simulink model "simpleMicrogrid_v1"  (R2020a)
settings: Solver=VariableStepAuto  StartTime=0.0  StopTime=24*60*60  RelTol=1e0
values from neighbouring files (symbols this model uses):
  to = 0.1    [v2gdata.mat]
  V2G =     [v2gdata.mat]
undefined symbols (not defined in the file or in its folder): A, B, C, Dd, Init, j, sigbuilder_block
libraries: simulink x28, powerlib x27, powerlib_meascontrol x5, simulink_extras x5, sps_avr x1, spsDieselMotorModel x1
(part 1 of 2)
settings Model: SimulationMode=accelerator  Creator=jlesage  LastModifiedBy=marko
settings DataIOCC: ReturnWorkspaceOutputs=off
settings DebuggingCC: UnconnectedInputMsg=none  UnconnectedOutputMsg=none  UnconnectedLineMsg=none  ArithmeticOperatorsInVariantConditions=warning
settings SFSimCC: SimUseLocalCustomCode=off  CustomCodeUndefinedFunction=UseInterfaceOnly
settings RTWCC: RTWUseLocalCustomCode=off

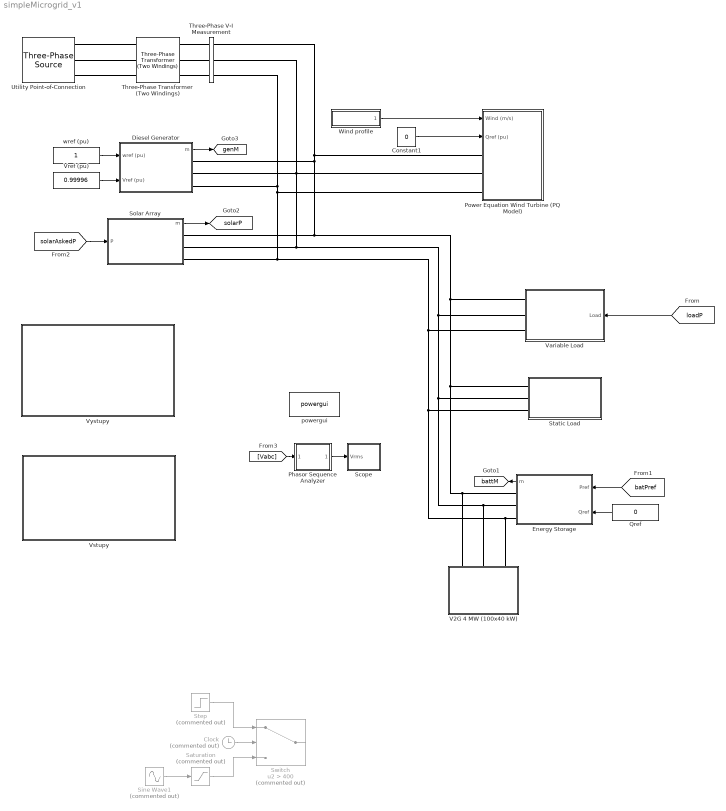
== system simpleMicrogrid_v1 ==
  Clock : Clock  Commented=on
  Constant1 : Constant  Value=0
  Diesel Generator : Subsystem  mask(Diesel Generator (Simple)){Pn=20e6, Vn=5000, Fn=60, genType=PQ, PQ0=[0.05 0]}
      mask prompts: Pn "Generator Rated Power [W]"; Vn "Rated Voltage [V]"; Fn "Rated Frequency [Hz]"; genType "Load Flow Type"; PQ0 "Initial Power, [P0 Q0] [pu]"
      mask help:
      | The Diesel Generator block contains a synchronous generator, diesel governor and excitation system to represent the dynamics of a Genset. To inspect the model, look under the block mask (Ctrl + u).
      |
      | The inputs to the basic Diesel generator block are the desired speed reference (in pu) and the desired voltage reference (in pu). The output measurements are contained in a Simulink bus, which can be selected by using the Bus Selector block.
      |
      | Note: The initial generator power must be specified for use for Load Flow analysis.
      mask init:
      | % Extract Initial Active/Reactive Power
      | P0 = PQ0(1);
      | Q0 = PQ0(2);
      | 
      | % Select Load Flow Type
      | genBlock = [gcb '/Synchronous Machine'];
      | currentVals = get_param(genBlock,'MaskValues');
      | currentVals{31} = genType;
      | set_param(genBlock,'MaskValues',currentVals);
      | 
      | % Disable Option if Swing Generator Selected
      | currentEnables = get_param(gcb,'MaskEnables');
      | if strcmp(genType,'swing')
      |     currentEnables{5} = 'off';
      | else
      |     currentEnables{5} = 'on';
      | end
      | set_param(gcb,'MaskEnables',currentEnables);
      settings: AttributesFormatString=Rated Power: %<Pn> W
      mask TypeOptions genType: swing | PQ | PV
      mask Display: %image(imread('diesel.jpg'))
  Energy Storage : Subsystem  mask(Grid-connected Energy Storage (PQ Model)){Vn=5000, Fn=60, PnomkW=5e5, kWh_Rated=1e5, Efficiency=96, LimitVec=[90 10], RechargeSOC=11, Precharge=50, autoRecharge=off, Initial_kWh_pc=80, PQvec=[100e3 0]}
      mask prompts: Vn "Nominal L-L Voltage [Vrms]"; Fn "Nominal Frequency [Hz]"; PnomkW "Rated Power [kW]"; kWh_Rated "Rated Capacity [kWh]"; Efficiency "Overall System Efficiency [%]"; LimitVec "Upper/Lower Charge Limits [%]"; RechargeSOC "SOC to Recharge [%]"; Precharge "Recharge Rate [% of Rated Power]"; autoRecharge "Enable Auto-Recharge"; Initial_kWh_pc "Initial State-of-Charge [0-100%]"; PQvec "Initial Active/Reactive Cmds"
      mask help:
      | The energy storage block models a generic grid-connected energy storage system (ESS), most commonly a battery system. This is a system-level model that does not contain any power electronics, but is useful for load flow, phasor, and hybrid phasor-EMT simulations. The inputs to this block are the commanded active and reactive power of the ESS. The ESS is assumed to have four quadrent operation.
      |
      | For more detailed ESS models, consider the battery block in the Drives library. Consider using this PQ Model to perform load flow studies and switch to a more detailed model when full EMT studies or more advanced controls are required.
      |
      | Note: The initial active/reactive power commands must be specified for use for Load Flow analysis.
      mask init:
      | % Calculate Initial Conditions
      | Pnom = PnomkW*1e3;
      | P0 = -PQvec(1);  Q0 = -PQvec(2);
      | if abs(P0) > Pnom
      |     P0 = sign(P0)*Pnom;
      | end
      | 
      | % Calculate Q0 given Reactive Power Capability Curve
      | Qlim = sqrt(Pnom^2 - P0^2);
      | if Qlim > abs(Q0)
      |     Q0 = sign(Q0)*Qlim;
      | end
      | 
      | UpChrgLim = LimitVec(1);
      | LowChrgLim = LimitVec(2);
      | if Initial_kWh_pc > UpChrgLim && P0 < 0
      |     P0 = 0; Q0 = 0;
      | elseif Initial_kWh_pc < LowChrgLim && P0 > 0
      |     P0 = 0; Q0 = 0;
      | end
      mask DialogControl Container7 Prompt: Grid Connection Properties
      mask DialogControl Container11 Prompt: Charge/Discharge Controls
      mask DialogControl Container12 Prompt: Initial Conditions
  Phasor Sequence Analyzer : Subsystem
  Power Equation Wind Turbine (PQ Model) : Subsystem  AncestorBlock=|  mask{Unom=15, Umax=25, Umin=5, Pselect=Simple Cubic Power, rp=5, Cp=16/27, rho=1.225, Pnom=500e3, Uvec=[1:1:30], Pvec=[0,0,0,0,21359.3750000000,58193.5000000000,104316.125000000,157104.500000000,213935.875000000,272187.500000000,329236.625000000,382460.500000000,429236.375000000,466941.500000000,492953.125000000,500000,500000,500000,500000,500000,500000,500000,500000,500000,500000,0,0,0,0,0], Tp=0.1, Tq=1, ReactP=30}
      | exampleMicrogridLibrary/Power Equation
      | Wind Turbine
      | (PQ Model)
      mask prompts: Unom "Nominal Wind Speed [m/s]"; Umax "Maximum Operating Wind [m/s]"; Umin "Minimum Operating Wind [m/s]"; Pselect "Wind Turbine Power Method"; rp "Blade Radius, r [m]"; Cp "Performance Coefficient, Cp"; rho "Air Density, rho [kg/m^3]"; Pnom "Nominal Power, [W]"; Uvec "Wind Vec [m/s]"; Pvec "Power Vec [W]"; Tp "Active Power Dynamics, Tp [s]"; Tq "Reactive Power Dynamics, Tq [s]"; ReactP "Reactive Power Percentage [%]"
      mask help:
      | Simple Wind Turbine that serves as an Active and Reactive Power Source depending on the Wind Power Curve.
      |
      | The Wind Turbine Power Curve can be defined by:
      | - Dimentions of the wind turbine
      | - Simple cubic power curve
      | - Look-up vector from a wind turbine data sheet.
      mask init:
      | A = pi*rp^2;
      | 
      | if Pselect == 1,
      |     Pmax = 1/2*rho*Cp*A*Umax^3;
      | elseif Pselect == 2,
      |     Pmax = Pnom;
      | else
      |     Pmax = max(Pvec);
      | end
      | Qmax = ReactP/100*Pmax;
      mask TypeOptions Pselect: Using Properties | Simple Cubic Power | Look-up Fit
      mask DialogControl Container4 Prompt: General
      mask DialogControl Container9 Prompt: Dimensions
      mask DialogControl Container12 Prompt: Cubic
      mask DialogControl Container7 Prompt: Lookup
      mask DialogControl Container8 Prompt: Dynamics
      mask Display:
      | image(imread('eolienne.bmp'))
      | 
      | color('white')
      | port_label('LConn',1,'A')
      | port_label('LConn',2,'B')
      | port_label('LConn',3,'C')
      | 
      | color('blue')
      | port_label('output',1,'m')
      | port_label('input',1,'Wind (m/s)')
      | port_label('input',2,'Qref')
  Qref : Constant  Value=0
  Saturation : Saturate  Commented=on  UpperLimit=15  LowerLimit=0
  Scope : Subsystem
  Sine Wave1 : Sin  Commented=on  Amplitude=20  Frequency=0.05  SampleTime=0
  Solar Array : Subsystem  mask(Grid-Connected PV Array (PQ Model)){Vn=5000, Fn=60, P0=500e3}
      mask prompts: Vn "Nominal L-L Voltage [Vrms]"; Fn "Nominal Frequency [Hz]"; P0 "Initial Power [W]"
      mask help:
      | This block models a grid-connected solar array using the Three-Phase Dynamic Load block. This is a system-level model that does not contain any power electronics, but is useful for load flow, phasor, and hybrid phasor-EMT simulations. The input to this block is the power output of the grid connected PV array, not irradiance.
      |
      | For more detailed PV models, consider the PV Array block in the Renewables library. Consider using this PQ Model to perform load flow studies and switch to a more detailed model when full EMT studies are required.
      |
      | Note: The array power must be specified for use for Load Flow analysis.
      mask init:
      | % P0 = Irr0*TotalArea*Efficiency/100;
      | P0 = -P0;
      mask Display:
      | image(imread('PV_Farm.jpg'))
      | color('white')
      | port_label('input',1,'P')
      | port_label('output',1,'m')
      | port_label('Rconn',1,'A')
      | port_label('Rconn',2,'B')
      | port_label('Rconn',3,'C')
  Static Load : Subsystem
  Step : Step  Commented=on  Time=550  Before=10  After=0  SampleTime=0
  Switch : Switch  Commented=on  Criteria=u2 > Threshold  Threshold=400
  Three-Phase Transformer (Two Windings) : powerlib/Elements/Three-Phase Transformer (Two Windings)  Winding1Connection=Yg  Winding2Connection=Yg  CoreType=Three single-phase transformers  SetSaturation=off  Hysteresis=off  DataFile='hysteresis'  SetInitialFlux=off  Measurements=None  UNITS=pu  NominalPower=[ 250e6 , 60 ]  Winding1=[ 13.8e3 , 0.002 , 0.08 ]  Winding2=[ 5000 , 0.002 , 0.08 ]  Rm=500  Lm=500  L0=0.5  Saturation=[ 0,0 ; 0.0024,1.2 ; 1.0,1.52 ]  InitialFluxes=[ 0.8 , -0.8 , 0.7 ]  BreakLoop=off  DiscreteSolver=Trapezoidal iterative  DataType=off  TransfoNumber=1
  Three-Phase V-I Measurement : powerlib/Measurements/Three-Phase V-I Measurement  VoltageMeasurement=phase-to-ground  SetLabelV=on  LabelV=Vabc  Vpu=off  VpuLL=off  CurrentMeasurement=yes  SetLabelI=on  LabelI=Iabc  Ipu=off  Pbase=100e6  Vbase=500e3  OutputType=Complex  PhasorSimulation=on  PSBequivalent=0
  Utility Point-of-Connection : powerlib/Electrical Sources/Three-Phase Source  InternalConnection=Yg  VoltagePhases=off  Voltage=(13800)*1.00293  PhaseAngle=0.16496  Voltage_phases=[25e3 25e3 25e3]/sqrt(3)  PhaseAngles_phases=[0 -120 +120]  Frequency=60  NonIdealSource=on  SpecifyImpedance=on  Resistance=0.8929  Inductance=16.58e-3  ShortCircuitLevel=250e6  BaseVoltage=13.8e3  XRratio=7  BusType=swing  Pref=10e3  Qref=0  Prefabc=[10e3, 10e3, 10e3]  Qrefabc=[0, 0, 0]  Qmin=-inf  Qmax=inf
  V2G 4 MW (100x40 kW) : Subsystem  mask{nomPower=20*2, capacity=85, eff=90, enable=on, regGain=[2 4e3], cars1=4, cars2=3, cars3=3, cars4=2, cars5=1}
      mask prompts: nomPower "Rated power (kW)"; capacity "Rated capacity (kWh)"; eff "System efficiency (%)"; enable "V2G on"; regGain "Regulator gain [Kp Ki]"; cars1 "Number of cars  (profile 1)"; cars2 "Number of cars  (profile 2)"; cars3 "Number of cars  (profile 3)"; cars4 "Number of cars  (profile 4)"; cars5 "Number of cars  (profile 5)"
      mask DialogControl DescGroupVar Prompt: V2G
      mask DialogControl DescTextVar Prompt: Models a generic aggregation of electric vehicles. The model has 5 different profiles that can be modified under the mask by changing the plug and the state of charge lookup tables of each profile. The user can set the number of vehicles following each type of profile. The rated capacity, the rated power and the efficiency of the power converter can also be decided by the user. See the example documentation for information about various user profiles.
      mask Display: image(imread('EV.jpg'))
  Variable Load : Subsystem  mask(Variable Load (PQ Model)){Vn=5000, Fn=60, PF=0.9500, Load0=200e3}
      mask prompts: Vn "Nominal L-L Voltage [Vrms]"; Fn "Nominal Frequency [Hz]"; PF "Power Factor [0 to 1]"; Load0 "Initial Load [W]"
      mask help:
      | The Variable Load block is a lumped approximation for a distribution feeder. For non-unity power factor loads, the input (active power) is scaled accordingly to generate a desired load.
      |
      | Note: The initial input load must be specified for use for Load Flow analysis.
      mask init:
      | P0 = Load0;
      | Q0 = Load0*sqrt(1/PF-1);
      mask Display:
      | image(imread('Residential.jpg'))
      | color('white')
      | port_label('input',1,'Load')
      | port_label('Rconn',1,'A')
      | port_label('Rconn',2,'B')
      | port_label('Rconn',3,'C')
  Vref (pu) : Constant  Value=0.99996
  Vstupy : Subsystem
  Vystupy : Subsystem
  Wind profile : Subsystem
      mask init:
      | load power_V2G
      mask Display: plot(V2G.WINDTURBINE.time,V2G.WINDTURBINE.wind)
  powergui : powerlib/powergui  Priority=1  SimulationMode=Phasor  SampleTime=1e-4  frequency=60  Iterations=50  frequencyindice=60  Pbase=100e6  ErrMax=1e-08  UnitsV=kV  UnitsW=MW  buscounter=6  FunctionMessages=off  echomessages=off  EnableUseOfTLC=off  CurrentSourceSwitches=off  DisableSnubberDevices=off  DisableRonSwitches=off  DisableVfSwitches=off  DisplayEquations=off  AutomaticDiscreteSolvers=off  SolverType=Tustin/Backward Euler (TBE)  Interpol=off  ExternalGateDelay=off  methode=off  Ts=100  x0status=blocks  SPID=on  SwTol=0  HookPort=off  NonlinearTolerance=1e-4  nMaxIteration=100  ContinueOnMaxIteration=off  RestoreLinks=warning  ResistiveCurrentMeasurement=off  Frange=[0:2:500]  Ylog=off  Xlog=on  ShowGrid=off  save=off  variable=ZData  structure=0  ZoomFFT=off  StartTime=0.0  cycles=1  DisplayStyle=1  fundamental=60  FreqAxis=off  MaxFrequency=1000  frequencyindicesteady=1  RmsSteady=1  display=off
  wref (pu) : Constant
  tag scope: battM=global, genM=global, solarP=global
  wires:
  Qref/1 -> Energy Storage/2(Qref)
  Energy Storage/1(m) -> [battM]
  Phasor Sequence Analyzer/1(Vrms) -> Scope/1(Vrms)
  [Vabc] -> Phasor Sequence Analyzer/1(Vabc)
  Step/1 -> Switch/1
  Sine Wave1/1 -> Saturation/1
  Saturation/1 -> Switch/3
  Clock/1 -> Switch/2
  wref (pu)/1 -> Diesel Generator/1(wref (pu))
  Diesel Generator/1(m) -> [genM]
  Vref (pu)/1 -> Diesel Generator/2(Vref (pu))
  Solar Array/1(m) -> [solarP]
  Wind profile/1(" ") -> Power Equation Wind Turbine (PQ Model)/1(Wind (m/s))
  Constant1/1 -> Power Equation Wind Turbine (PQ Model)/2(Qref (pu))
  [loadP] -> Variable Load/1(Load)
  [solarAskedP] -> Solar Array/1(P)
  [batPref] -> Energy Storage/1(Pref)
  connections:
  Diesel Generator/RConn2 -- Static Load/LConn2 -- Energy Storage/RConn2 -- V2G 4 MW (100x40 kW)/LConn2 -- Variable Load/RConn2 -- Solar Array/RConn2 -- Power Equation Wind Turbine (PQ Model)/LConn2 -- Three-Phase V-I Measurement/RConn2
  Energy Storage/RConn1 -- V2G 4 MW (100x40 kW)/LConn1 -- Static Load/LConn1 -- Variable Load/RConn1 -- Three-Phase V-I Measurement/RConn1 -- Power Equation Wind Turbine (PQ Model)/LConn1 -- Diesel Generator/RConn1 -- Solar Array/RConn1
  Energy Storage/RConn3 -- V2G 4 MW (100x40 kW)/LConn3 -- Static Load/LConn3 -- Variable Load/RConn3 -- Solar Array/RConn3 -- Three-Phase V-I Measurement/RConn3 -- Diesel Generator/RConn3 -- Power Equation Wind Turbine (PQ Model)/LConn3
  Three-Phase Transformer (Two Windings)/RConn3 -- Three-Phase V-I Measurement/LConn3
  Three-Phase Transformer (Two Windings)/RConn2 -- Three-Phase V-I Measurement/LConn2
  Three-Phase Transformer (Two Windings)/RConn1 -- Three-Phase V-I Measurement/LConn1
  Utility Point-of-Connection/RConn1 -- Three-Phase Transformer (Two Windings)/LConn1
  Utility Point-of-Connection/RConn2 -- Three-Phase Transformer (Two Windings)/LConn2
  Utility Point-of-Connection/RConn3 -- Three-Phase Transformer (Two Windings)/LConn3

== system simpleMicrogrid_v1/Diesel Generator ==
  wref (pu) : Inport
  Vref (pu) : Inport  Port=2
  AC1A Excitation System : sps_avr/AC1A Excitation System  Tr=20e-3  KaTa=[400 0.02]  VAminmax=[-14.5 14.5]  VRminmax=[-5.43 6.03]  KfTf=[0.03 1.0]  TbTc=[0 0]  KeTe=[1.0 0.80]  Ve12=[4.18 3.14]  SeVe12=[0.10 0.03]  Kd=0.38  Kc=0.20  v0=[0.99996 1.0014]  TsBlock=0
      settings: SourceProductBaseCode=PS
  Diesel Engine Governor : spsDieselMotorModel/Diesel Engine Governor  K=29  Tr=[0.01 0.02 0.2]  Ta=[0.25 0.009 0.0384]  Tlim=[0 1.1]  Td=0.024  Pm0=0.050008
      settings: SourceProductBaseCode=PS
  Generator Measures : Subsystem
  Ground : Ground
  Selected Measurements : Subsystem
  Synchronous Machine : powerlib/Machines/Synchronous Machine pu Standard  PresetModel=No  MechanicalLoad=Mechanical power Pm  ShowDetailedParameters=on  RotorType=Salient-pole  Units=per unit standard parameters  MeasurementBus=off  NominalParameters=[ Pn Vn Fn]  Reactances1=[ 1.81, 0.3, 0.23, 1.76, 0.65, 0.25, 0.15 ]  Reactances2="[ 1.305, 0.296, 0.252, 0.474,  0.243,  0.18 ]"  dAxisTimeConstants=Open-circuit  qAxisTimeConstants=Short-circuit  TimeConstants1="[ 4.4849  0.0681  0.1  ]"  TimeConstants2=[ 8.0, 0.03, 1.0, 0.07 ]  TimeConstants3="[  4.49  0.0681  0.0513  ]"  TimeConstants4=[ 8.0, 0.03, 0.3371, 0.0295 ]  TimeConstants5=[ 1.01, 0.053, 0.1 ]  TimeConstants6=[ 1.3201, 0.023, 1.0, 0.07 ]  TimeConstants7=[0.012 0.003 0.003]  TimeConstants8=[ 1.3201, 0.0231, 0.3371, 0.0295 ]  StatorResistance=0.003  Mechanical=[3.7 0 1 ]  PolePairs=20  InitialConditions=[0 -88.6613 0.0500019 0.0500019 0.0500019 -0.018842 -120.019 119.981 1.00138]  SetSaturation=off  Saturation=[0.6404,0.7127,0.8441,0.9214,0.9956,1.082,1.19,1.316,1.457;0.7,0.7698,0.8872,0.9466,0.9969,1.046,1.1,1.151,1.201]  LoadFlowParameters=[1,0,0,0,0]  TsPowergui=0  TsBlock=-1  IterativeModel=Trapezoidal non iterative  IterativeDiscreteModel=Trapezoidal non iterative  BusType=PQ  Pref=Pn*P0  Qref=0  Qmin=-inf  Qmax=inf  PLF=0  QLF=0
  A : PMIOPort  Side=Right
  B : PMIOPort  Port=2  Side=Right
  C : PMIOPort  Port=3  Side=Right
  m : Outport  VectorParamsAs1DForOutWhenUnconnected=off
  wires:
  wref (pu)/1 -> Diesel Engine Governor/1
  Vref (pu)/1 -> AC1A Excitation System/1
  Synchronous Machine/1 -> Generator Measures/1(m), Selected Measurements/1(m)
  Ground/1 -> AC1A Excitation System/4
  Generator Measures/3(wm) -> Diesel Engine Governor/2
  Generator Measures/2(Vt) -> AC1A Excitation System/2
  Generator Measures/1(Ifd) -> AC1A Excitation System/3
  Selected Measurements/1(sm) -> m/1
  Diesel Engine Governor/1 -> Synchronous Machine/1
  AC1A Excitation System/1 -> Synchronous Machine/2
  connections:
  Synchronous Machine/RConn1 -- A/RConn1
  Synchronous Machine/RConn3 -- C/RConn1
  Synchronous Machine/RConn2 -- B/RConn1

== system simpleMicrogrid_v1/Energy Storage ==
  Pref : Inport
  Qref : Inport  Port=2
  Bus Creator : BusCreator  Inputs=3
  Charge Limits : Subsystem
  Mux1 : Mux  Inputs=2
  Power Limits : Saturate  UpperLimit=Pnom  LowerLimit=-Pnom
  Reactive Power Capability : Subsystem
  Simple Battery Inverter : powerlib/Elements/Three-Phase Dynamic Load  NominalVoltage=[Vn Fn]  ActiveReactivePowers=[-100000 -3.07049e-13]  PositiveSequence=[0.999962 -0.018842]  ExternalControl=on  NpNq=[1.3 2]  TimeConstants="[0  0  0  0]"  MinimumVoltage=0.7  Tfilter=1e-2  LoadFlowParameters=[4,0,0,0,0]
      settings: SourceProductBaseCode=PS
  Stored Energy Calculation (%) : Subsystem
  Terminator : Terminator
  Unary Minus : UnaryMinus
  A : PMIOPort  Side=Right
  B : PMIOPort  Port=2  Side=Right
  C : PMIOPort  Port=3  Side=Right
  m : Outport  VectorParamsAs1DForOutWhenUnconnected=off
  wires:
  Charge Limits/2(Qbatt) -> Reactive Power Capability/2(Qin)
  Qref/1 -> Charge Limits/3(Qin)
  Power Limits/1 -> Charge Limits/2(Pin)
  Charge Limits/1(Pbatt) -> Reactive Power Capability/1(Pin), Unary Minus/1, Bus Creator/2, Stored Energy Calculation (%)/1(Pin)  "Pbatt"
  Stored Energy Calculation (%)/1(SE%) -> Bus Creator/1, Charge Limits/1(SOC (%))  "SOC (%)"
  Bus Creator/1 -> m/1
  Pref/1 -> Power Limits/1
  Reactive Power Capability/1(Qout) -> Mux1/2, Bus Creator/3, Stored Energy Calculation (%)/2(Qin)  "Qbatt"
  Simple Battery Inverter/1 -> Terminator/1
  Mux1/1 -> Simple Battery Inverter/1
  Unary Minus/1 -> Mux1/1
  connections:
  Simple Battery Inverter/LConn1 -- A/RConn1
  Simple Battery Inverter/LConn3 -- C/RConn1
  Simple Battery Inverter/LConn2 -- B/RConn1

== system simpleMicrogrid_v1/Phasor Sequence Analyzer ==
  Vabc : Inport
  Sequence Analyzer (Phasor) : powerlib_meascontrol/Measurements/Sequence Analyzer (Phasor)  seq=Positive
      settings: SourceProductBaseCode=PS
  Terminator : Terminator
  Vrms : Outport  VectorParamsAs1DForOutWhenUnconnected=off
  wires:
  Sequence Analyzer (Phasor)/1 -> Vrms/1
  Vabc/1 -> Sequence Analyzer (Phasor)/1
  Sequence Analyzer (Phasor)/2 -> Terminator/1

== system simpleMicrogrid_v1/Power Equation Wind Turbine (PQ Model) ==
  Wind (m/s) : Inport
  Qref (pu) : Inport  Port=2
  Active Power Dynamics : Subsystem  VariantControl=T6NotZero
      mask Display: disp('1 / (1 + s T_P)','texmode','on');
  Bus Selector : BusSelector  OutputSignals=Active power P (W)
  Ground : powerlib/Elements/Ground  LConnTagsString=a
  Mux : Mux  Inputs=2
  Reactive Power Dynamics : Subsystem  VariantControl=T6NotZero
      mask Display: disp('1 / (1 + s T_Q)','texmode','on');
  Saturation : Saturate  UpperLimit=Qmax  LowerLimit=-Qmax
  Scope1 : Scope
  Shunt (Numerical Stability) : powerlib/Elements/Three-Phase Series RLC Branch  LConnTagsString=A|B|C  RConnTagsString=A|B|C  BranchType=R  Resistance=1e9  Inductance=1e-3  Capacitance=1e-6  Measurements=None
  Three-Phase Dynamic Load : powerlib/Elements/Three-Phase Dynamic Load  NominalVoltage=[5000 60]  ActiveReactivePowers=[50e6 25e6]  PositiveSequence=[0.994 -11.8]  ExternalControl=on  NpNq=[1.3 2]  TimeConstants="[0  0  0  0]"  MinimumVoltage=0.7  Tfilter=1e-4  LoadFlowParameters=[4,0,0,0,0]
      settings: SourceProductBaseCode=PS
  Wind Turbine Power Equation : Subsystem
  A : PMIOPort  Side=Left
  B : PMIOPort  Port=2  Side=Left
  C : PMIOPort  Port=3  Side=Left
  tag scope: windP=global
  wires:
  Qref (pu)/1 -> Saturation/1
  Saturation/1 -> Reactive Power Dynamics/1(In)
  Reactive Power Dynamics/1(Out) -> Mux/2
  Active Power Dynamics/1(Out) -> Mux/1
  Mux/1 -> Three-Phase Dynamic Load/1
  Wind Turbine Power Equation/1(Pwind) -> Active Power Dynamics/1(In)
  Wind (m/s)/1 -> Wind Turbine Power Equation/1(Wind (m/s))
  Bus Selector/1 -> Scope1/1, [windP]  "<Active power P (W)>"
  Three-Phase Dynamic Load/1 -> Bus Selector/1
  connections:
  Ground/LConn1 -- Shunt (Numerical Stability)/RConn1 -- Shunt (Numerical Stability)/RConn2 -- Shunt (Numerical Stability)/RConn3
  Shunt (Numerical Stability)/LConn1 -- Three-Phase Dynamic Load/LConn1 -- A/RConn1
  Shunt (Numerical Stability)/LConn3 -- Three-Phase Dynamic Load/LConn3 -- C/RConn1
  Shunt (Numerical Stability)/LConn2 -- Three-Phase Dynamic Load/LConn2 -- B/RConn1

== system simpleMicrogrid_v1/Scope ==
  Vrms : Inport
  Bus Selector1 : BusSelector  OutputSignals=SOC (%)  OutputAsBus=on
  Bus Selector2 : BusSelector  OutputSignals=Pbatt
  Bus Selector3 : BusSelector  OutputSignals=Active Power (W)
  Bus Selector4 : BusSelector  OutputSignals="Rotor speed  wm  (pu)"
  Gain : Gain  Gain=60
  LG to LL : Gain  Gain=sqrt(3)/sqrt(2)
  Microgrid Measures : Scope  NumInputPorts=4
  Mux : Mux
  Scope : Scope
  to kW : Gain  Gain=1e-3
  wires:
  Bus Selector3/1 -> Mux/4  "<Active Power (W)>"
  to kW/1 -> Scope/1, Microgrid Measures/2  "Distributed Resources (kW)"
  Bus Selector4/1 -> Gain/1  "<Rotor speed  wm  (pu)>"
  [genM] -> Bus Selector4/1
  Gain/1 -> Microgrid Measures/1  "Microgrid Frequency (Hz)"
  Bus Selector1/1 -> Microgrid Measures/3  "Battery SOC (%)"
  [battM] -> Bus Selector1/1
  [genM] -> Bus Selector3/1
  [battM] -> Bus Selector2/1
  Bus Selector2/1 -> Mux/3  "<Pbatt>"
  [solarP] -> Mux/2
  Mux/1 -> to kW/1
  LG to LL/1 -> Microgrid Measures/4  "Microgrid Voltage (Vrms)"
  Vrms/1 -> LG to LL/1
  [windP] -> Mux/1

== system simpleMicrogrid_v1/Solar Array ==
  P : Inport
  Bus Selector : BusSelector  OutputSignals=Active power P (W)
  Constant11 : Constant  Value=0
  Mux1 : Mux  Inputs=2
  Simple Solar Inverter : powerlib/Elements/Three-Phase Dynamic Load  NominalVoltage=[Vn Fn]  ActiveReactivePowers=[-250000 -2.85874e-13]  PositiveSequence=[0.999962 -0.018842]  ExternalControl=on  NpNq=[1.3 2]  TimeConstants="[0  0  0  0]"  MinimumVoltage=0.7  Tfilter=1e-2  LoadFlowParameters=[4,0,0,0,0]
      settings: SourceProductBaseCode=PS
  Unary Minus : UnaryMinus
  Unary Minus1 : UnaryMinus
  A : PMIOPort  Side=Right
  B : PMIOPort  Port=2  Side=Right
  C : PMIOPort  Port=3  Side=Right
  m : Outport  VectorParamsAs1DForOutWhenUnconnected=off
  wires:
  P/1 -> Unary Minus/1
  Unary Minus/1 -> Mux1/1
  Constant11/1 -> Mux1/2
  Simple Solar Inverter/1 -> Bus Selector/1
  Bus Selector/1 -> Unary Minus1/1  "<Active power P (W)>"
  Unary Minus1/1 -> m/1
  Mux1/1 -> Simple Solar Inverter/1
  connections:
  Simple Solar Inverter/LConn2 -- B/RConn1
  Simple Solar Inverter/LConn3 -- C/RConn1
  Simple Solar Inverter/LConn1 -- A/RConn1

== system simpleMicrogrid_v1/Static Load ==
  Load : powerlib/Elements/Three-Phase Series RLC Load  LConnTagsString=A|B|C  Configuration=Y (grounded)  NominalVoltage=(5000)*0.999962  Vabc=[1e3 1e3 1e3]  Vabcp=[1e3 1e3 1e3]  NominalFrequency=60  UnbalancedPower=off  ActivePower=500e3  InductivePower=0  CapacitivePower=0  Pabc=[10e3 9e3 11e3]  QLabc=[100 90 110]  QCabc=[100 90 110]  Pabcp=[10e3 9e3 11e3]  QLabcp=[100 90 110]  QCabcp=[100 90 110]  Measurements=Branch voltages  LoadType=constant PQ
      settings: AttributesFormatString=P = %<ActivePower> W
  "Power (3ph, Phasor)5" : powerlib_meascontrol/Measurements/Power (3ph, Phasor)
      settings: SourceProductBaseCode=MT,PS
  Scope : Scope
  Terminator : Terminator
  Three-Phase V-I Measurement : powerlib/Measurements/Three-Phase V-I Measurement  VoltageMeasurement=phase-to-ground  SetLabelV=on  LabelV=VabcLoad  Vpu=off  VpuLL=off  CurrentMeasurement=yes  SetLabelI=on  LabelI=IabcLoad  Ipu=off  Pbase=100e6  Vbase=500e3  OutputType=Complex  PhasorSimulation=on  PSBequivalent=0
  A : PMIOPort  Side=Left
  B : PMIOPort  Port=2  Side=Left
  C : PMIOPort  Port=3  Side=Left
  tag scope: PLoad=global
  wires:
  [VabcLoad] -> "Power (3ph, Phasor)5"/1
  [IabcLoad] -> "Power (3ph, Phasor)5"/2
  "Power (3ph, Phasor)5"/2 -> Terminator/1  "Q(VA)"
  "Power (3ph, Phasor)5"/1 -> Scope/1, [PLoad]  "P(W)"
  connections:
  Load/LConn1 -- Three-Phase V-I Measurement/RConn1
  Load/LConn2 -- Three-Phase V-I Measurement/RConn2
  Load/LConn3 -- Three-Phase V-I Measurement/RConn3
  Three-Phase V-I Measurement/LConn1 -- A/RConn1
  B/RConn1 -- Three-Phase V-I Measurement/LConn2
  Three-Phase V-I Measurement/LConn3 -- C/RConn1

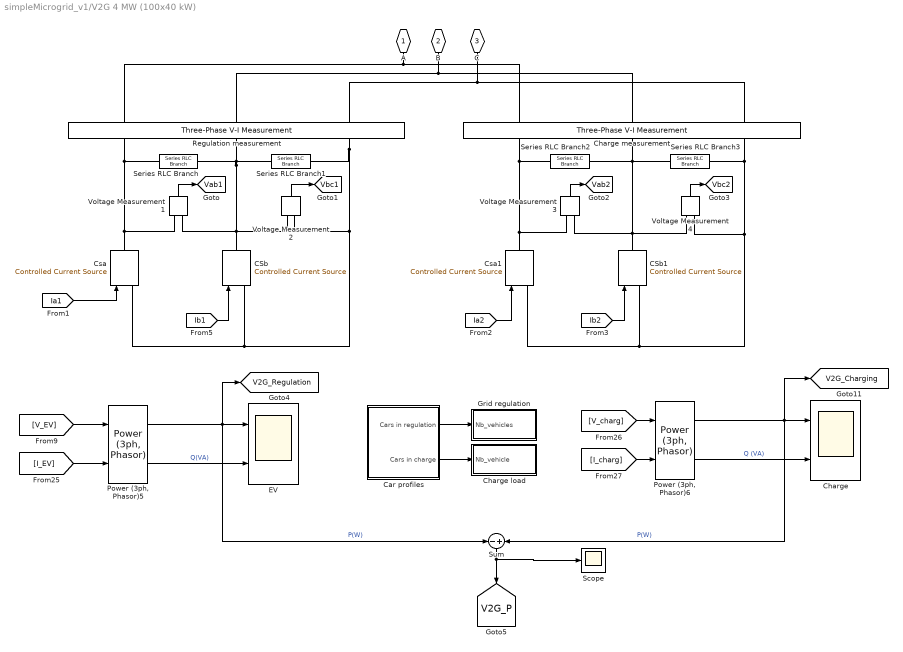
== system simpleMicrogrid_v1/V2G 4 MW (100x40 kW) ==
  " Charge measurement" : powerlib/Measurements/Three-Phase V-I Measurement  VoltageMeasurement=phase-to-ground  SetLabelV=on  LabelV=V_charg  Vpu=off  VpuLL=off  CurrentMeasurement=yes  SetLabelI=on  LabelI=I_charg  Ipu=off  Pbase=2*1.5e6/0.9  Vbase=25e3  OutputType=Complex  PhasorSimulation=on  PSBequivalent=0
      settings: SourceProductBaseCode=MT,PS
  " Regulation measurement" : powerlib/Measurements/Three-Phase V-I Measurement  VoltageMeasurement=phase-to-ground  SetLabelV=on  LabelV=V_EV  Vpu=off  VpuLL=off  CurrentMeasurement=yes  SetLabelI=on  LabelI=I_EV  Ipu=off  Pbase=2*1.5e6/0.9  Vbase=25e3  OutputType=Complex  PhasorSimulation=on  PSBequivalent=0
      settings: SourceProductBaseCode=MT,PS
  CSb : powerlib/Electrical Sources/Controlled Current Source  Initialize=on  Source_Type=AC  Amplitude=5604.181  Phase=(2.761-2*pi/3)*180/pi  Frequency=60  Measurements=Current
      settings: SourceProductBaseCode=MT,PS
  CSb1 : powerlib/Electrical Sources/Controlled Current Source  Initialize=on  Source_Type=AC  Amplitude=5604.181  Phase=(2.761-2*pi/3)*180/pi  Frequency=60  Measurements=Current
      settings: SourceProductBaseCode=MT,PS
  Car profiles : Subsystem
  Charge : Scope  NumInputPorts=2
  Charge load : Subsystem
  Csa : powerlib/Electrical Sources/Controlled Current Source  Initialize=on  Source_Type=AC  Amplitude=5604.181  Phase=2.761*180/pi  Frequency=60  Measurements=Current
      settings: SourceProductBaseCode=MT,PS
  Csa1 : powerlib/Electrical Sources/Controlled Current Source  Initialize=on  Source_Type=AC  Amplitude=5604.181  Phase=2.761*180/pi  Frequency=60  Measurements=Current
      settings: SourceProductBaseCode=MT,PS
  EV : Scope  NumInputPorts=2
  Grid regulation : Subsystem
  "Power (3ph, Phasor)5" : powerlib_meascontrol/Measurements/Power (3ph, Phasor)
      settings: SourceProductBaseCode=MT,PS
  "Power (3ph, Phasor)6" : powerlib_meascontrol/Measurements/Power (3ph, Phasor)
      settings: SourceProductBaseCode=MT,PS
  Scope : Scope
  Series RLC Branch{,1..3} (4 alike) : powerlib/Elements/Series RLC Branch  LConnTagsString=__new0  RConnTagsString=__new0  BranchType=R  Resistance=1e6  Inductance=1e-3  SetiL0=off  InitialCurrent=0  Capacitance=1e-6  Setx0=off  InitialVoltage=0  Measurements=None
      settings: SourceProductBaseCode=MT,PS
  Sum : Sum  Inputs=-+
  Voltage Measurement{1..4} (4 alike) : powerlib/Measurements/Voltage Measurement  PhasorSimulation=on  OutputType=Complex  PSBequivalent=0
      settings: SourceProductBaseCode=MT,PS
  "A " : PMIOPort  Tag=PMCPort  Side=Left
  B : PMIOPort  Tag=PMCPort  Port=2  Side=Left
  "C " : PMIOPort  Tag=PMCPort  Port=3  Side=Left
  tag scope: V2G_Charging=global, V2G_P=global, V2G_Regulation=global, Vab1=global, Vab2=global, Vbc1=global, Vbc2=global
  wires:
  Voltage Measurement1/1 -> [Vab1]
  Voltage Measurement2/1 -> [Vbc1]
  [Ia1] -> Csa/1
  [Ib1] -> CSb/1
  Voltage Measurement3/1 -> [Vab2]
  Voltage Measurement4/1 -> [Vbc2]
  [Ia2] -> Csa1/1
  [Ib2] -> CSb1/1
  Car profiles/1(Cars in regulation) -> Grid regulation/1(Nb_vehicles)
  Car profiles/2(" Cars in charge") -> Charge load/1(Nb_vehicle)
  [I_EV] -> "Power (3ph, Phasor)5"/2
  [V_charg] -> "Power (3ph, Phasor)6"/1
  [I_charg] -> "Power (3ph, Phasor)6"/2
  [V_EV] -> "Power (3ph, Phasor)5"/1
  "Power (3ph, Phasor)6"/1 -> Sum/2, [V2G_Charging], Charge/1  "P(W)"
  "Power (3ph, Phasor)6"/2 -> Charge/2  "Q (VA)"
  "Power (3ph, Phasor)5"/1 -> Sum/1, [V2G_Regulation], EV/1  "P(W)"
  "Power (3ph, Phasor)5"/2 -> EV/2  "Q(VA)"
  Sum/1 -> Scope/1, [V2G_P]
  connections:
  Series RLC Branch/LConn1 -- Csa/RConn1 -- Voltage Measurement1/LConn1 -- " Regulation measurement"/LConn1
  Voltage Measurement2/LConn2 -- Series RLC Branch1/RConn1 -- " Regulation measurement"/LConn3 -- Csa/LConn1 -- CSb/LConn1
  Voltage Measurement1/LConn2 -- " Regulation measurement"/LConn2 -- Series RLC Branch1/LConn1 -- Series RLC Branch/RConn1 -- CSb/RConn1 -- Voltage Measurement2/LConn1
  Voltage Measurement3/LConn1 -- Csa1/RConn1 -- Series RLC Branch2/LConn1 -- " Charge measurement"/RConn1
  Series RLC Branch3/RConn1 -- Csa1/LConn1 -- CSb1/LConn1 -- Voltage Measurement4/LConn2 -- " Charge measurement"/RConn3
  Series RLC Branch3/LConn1 -- Series RLC Branch2/RConn1 -- CSb1/RConn1 -- Voltage Measurement4/LConn1 -- Voltage Measurement3/LConn2 -- " Charge measurement"/RConn2
  " Regulation measurement"/RConn1 -- " Charge measurement"/LConn1 -- "A "/RConn1
  " Regulation measurement"/RConn2 -- " Charge measurement"/LConn2 -- B/RConn1
  " Regulation measurement"/RConn3 -- " Charge measurement"/LConn3 -- "C "/RConn1

== system simpleMicrogrid_v1/Variable Load ==
  Load : Inport
  Bus Selector : BusSelector  OutputSignals=Active power P (W)
  Dynamic Load Control : Subsystem
  Scope : Scope
  Simple Three-Phase Load : powerlib/Elements/Three-Phase Dynamic Load  NominalVoltage=[Vn Fn]  ActiveReactivePowers=[200000 45883.1]  PositiveSequence=[0.999962 -0.018842]  ExternalControl=on  NpNq=[1.3 2]  TimeConstants="[0  0  0  0]"  MinimumVoltage=0.7  Tfilter=1e-2  LoadFlowParameters=[4,0,0,0,0]
      settings: SourceProductBaseCode=PS
  A : PMIOPort  Side=Right
  B : PMIOPort  Port=2  Side=Right
  C : PMIOPort  Port=3  Side=Right
  tag scope: varLoadP=global
  wires:
  Simple Three-Phase Load/1 -> Bus Selector/1
  Load/1 -> Dynamic Load Control/1(P0)
  Dynamic Load Control/1(PQ) -> Scope/1, Simple Three-Phase Load/1
  Bus Selector/1 -> [varLoadP]  "<Active power P (W)>"
  connections:
  Simple Three-Phase Load/LConn1 -- A/RConn1
  Simple Three-Phase Load/LConn3 -- C/RConn1
  Simple Three-Phase Load/LConn2 -- B/RConn1

== system simpleMicrogrid_v1/Vstupy ==
  Add : Sum
  Bateria : Subsystem  Tag=STV Subsys  Commented=on  LoadFcn=sigbuilder_block('load');  StartFcn=sigbuilder_block('start');  StopFcn=sigbuilder_block('stop');  ClipboardFcn=sigbuilder_block('clipboard');  mask(Sigbuilder block){tuvar=[0:10]}
      mask help: Simulink:masks:SigbuilderBlock_MD
      mask init:
      | if ~strcmp(get_param(bdroot(gcbh),'SimulationStatus'),'stopped') tuvar = sigbuilder_block('maskInit'); end
      settings: CopyFcn=sigbuilder_block('copy');  DeleteFcn=sigbuilder_block('delete');  ModelCloseFcn=sigbuilder_block('modelClose');  PreSaveFcn=sigbuilder_block('preSave');  PauseFcn=sigbuilder_block('pause');  ContinueFcn=sigbuilder_block('continue');  NameChangeFcn=sigbuilder_block('namechange');  OpenFcn=sigbuilder_block('open',[437.6 199.2 550.4 400 ]);  CloseFcn=sigbuilder_block('close');
      mask Display: plot(0, 0, 100, 100,[2, 2, 32, 32, 2], [68, 8, 8, 68, 68],[32, 2], [38, 38], [32, 19, 2],[53, 60, 44], [32, 17, 17, 2],[16, 16, 31, 31]);txt = getActiveGroup(gcbh);text(2, 100, txt,'verticalAlignment', 'top');
  Clock1 : Clock
  Constant : Constant
  Gain : Gain  Gain=10e5
  Gain1 : Gain  Gain=1e3
  Goto1 : Goto  Commented=on  GotoTag=batPref  TagVisibility=global
  Irradiance : Subsystem
      mask init:
      | load power_V2G
      mask Display: plot(V2G.IRRADIANCE.time,V2G.IRRADIANCE.SUN)
  Partial Shading : Subsystem  mask(Signal Disturbance){Hour=12, Minute=0, Second=0, Duration=5*60, Factor=0.7}
      mask prompts: Duration "Duration (s):"
      mask help: Within the specified time range defined by Start and Duration parameters, output is set to 'Factor'. Outside the specified time range output is kept at 1.0.
      mask init:
      | T2=(Hour-1)*60*60;    % Hour in seconds
      | T3=(Minute-1)*60;  % Minute in seconds
      | Ton=T2+T3+(Second-1);    % Beginning of fault (s)
      | Toff=Ton+Duration; % End of fault (s)
      mask TypeOptions Hour: 0 |      1 |      2 |      3 |      4 |      5 |      6 |      7 |      8 |      9 |     10 |     11 |     12 |     13 |     14 |     15 |     16 |     17 |     18 |     19 |     20 |     21 |     22 |     23
      mask TypeOptions Minute: 0 |      1 |      2 |      3 |      4 |      5 |      6 |      7 |      8 |      9 |     10 |     11 |     12 |     13 |     14 |     15 |     16 |     17 |     18 |     19 |     20 |     21 |     22 |     23 |     24 |     25 |     26 |     27 |     28 |     29 |     30 |     31 |     32 |     33 |     34 |     35 |     36 |     37 |     38 |     39 |     40 |     41 |     42 |     43 |     44 |     45 |     46 |     47 |     48 |     49 |     50 |     51 |     52 |     53 |     54 |     55 |     56 |     57 |     58 |     59
      mask TypeOptions Second: 0 |      1 |      2 |      3 |      4 |      5 |      6 |      7 |      8 |      9 |     10 |     11 |     12 |     13 |     14 |     15 |     16 |     17 |     18 |     19 |     20 |     21 |     22 |     23 |     24 |     25 |     26 |     27 |     28 |     29 |     30 |     31 |     32 |     33 |     34 |     35 |     36 |     37 |     38 |     39 |     40 |     41 |     42 |     43 |     44 |     45 |     46 |     47 |     48 |     49 |     50 |     51 |     52 |     53 |     54 |     55 |     56 |     57 |     58 |     59
      mask DialogControl Control2 Prompt: Start:
  Power consumption : Lookup_n-D  NumberOfTableDimensions=1  BreakpointsForDimension1=[1:24]  BeginIndexSearchUsingPreviousIndexResult=on  Table=V2G.CONSUMPTION  InternalRulePriority=Speed  RndMeth=Simplest  InputSameDT=on
  Product1 : Product
  Random Number : RandomNumber  Commented=on  Mean=-1e5  Variance=2e5  Seed=1  SampleTime=1000
  Rate Limiter2 : RateLimiter  RisingSlewLimit=1e4  FallingSlewLimit=-1e4  SampleTimeMode=inherited
  Scope : Scope  Commented=on
  Scope1 : Scope
  Scope3 : Scope
  Second-->Hour : Gain  Gain=1/(60*60)
  tag scope: loadP=global, solarAskedP=global
  wires:
  Bateria/1(Signal 1) -> Goto1/1
  Power consumption/1 -> Gain/1
  Constant/1 -> Add/2
  Second-->Hour/1 -> Add/1
  Add/1 -> Power consumption/1
  Gain/1 -> [loadP], Scope3/1
  Clock1/1 -> Second-->Hour/1
  Random Number/1 -> Scope/1
  Partial Shading/1(Out) -> Product1/2
  Irradiance/1(" ") -> Product1/1
  Rate Limiter2/1 -> Gain1/1
  Product1/1 -> Rate Limiter2/1
  Gain1/1 -> Scope1/1, [solarAskedP]

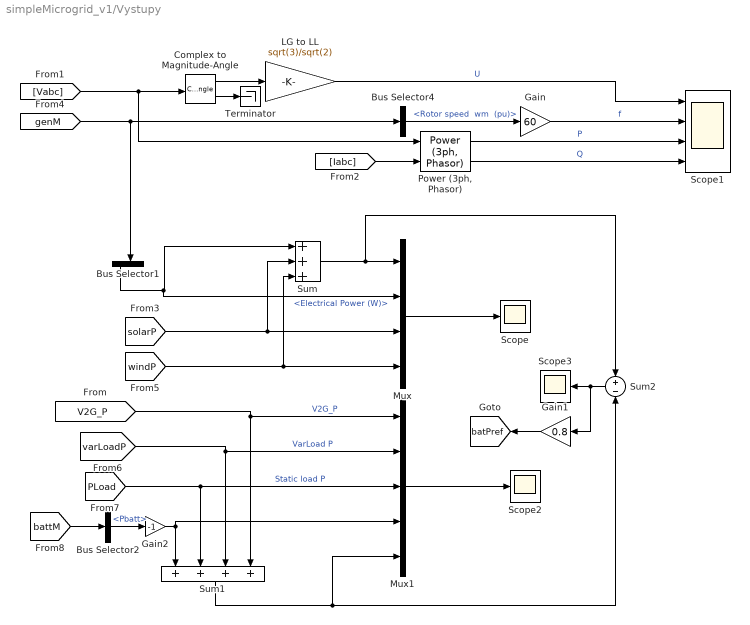
== system simpleMicrogrid_v1/Vystupy ==
  Bus Selector1 : BusSelector  OutputSignals=Electrical Power (W),Active Power (W)
  Bus Selector2 : BusSelector  OutputSignals=Pbatt
  Bus Selector4 : BusSelector  OutputSignals="Rotor speed  wm  (pu)"
  Complex to Magnitude-Angle : ComplexToMagnitudeAngle
  Gain : Gain  Gain=60
  Gain1 : Gain  Gain=0.8
  Gain2 : Gain  Gain=-1
  LG to LL : Gain  Gain=sqrt(3)/sqrt(2)
  Mux : Mux
  Mux1 : Mux  Inputs=5
  "Power (3ph, Phasor)" : powerlib_meascontrol/Measurements/Power (3ph, Phasor)
      settings: SourceProductBaseCode=PS
  Scope : Scope
  Scope1 : Scope  NumInputPorts=4
  Scope2 : Scope
  Scope3 : Scope
  Sum : Sum  Inputs=+++
  Sum1 : Sum  Inputs=++++
  Sum2 : Sum  Inputs=+-
  Terminator : Terminator
  tag scope: batPref=global
  wires:
  Bus Selector4/1 -> Gain/1  "<Rotor speed  wm  (pu)>"
  Complex to Magnitude-Angle/1 -> LG to LL/1
  [Iabc] -> "Power (3ph, Phasor)"/2
  Complex to Magnitude-Angle/2 -> Terminator/1
  "Power (3ph, Phasor)"/2 -> Scope1/4  "Q"
  [Vabc] -> Complex to Magnitude-Angle/1, "Power (3ph, Phasor)"/1
  "Power (3ph, Phasor)"/1 -> Scope1/3  "P"
  [genM] -> Bus Selector1/1, Bus Selector4/1
  Gain/1 -> Scope1/2  "f"
  LG to LL/1 -> Scope1/1  "U"
  [solarP] -> Sum/2, Mux/3
  [windP] -> Mux/4, Sum/3
  Sum/1 -> Sum2/1, Mux/1
  Mux/1 -> Scope/1
  [PLoad] -> Sum1/2, Mux1/3  "Static load P"
  [varLoadP] -> Mux1/2, Sum1/3  "VarLoad P"
  Sum1/1 -> Sum2/2, Mux1/5
  Mux1/1 -> Scope2/1
  [battM] -> Bus Selector2/1
  Bus Selector2/1 -> Gain2/1  "<Pbatt>"
  Bus Selector1/1 -> Mux/2, Sum/1  "<Electrical Power (W)>"
  [V2G_P] -> Mux1/1, Sum1/4  "V2G_P"
  Sum2/1 -> Gain1/1, Scope3/1
  Gain2/1 -> Sum1/1, Mux1/4
  Gain1/1 -> [batPref]

== system simpleMicrogrid_v1/Wind profile ==
  1-D Lookup Table : Lookup_n-D  NumberOfTableDimensions=1  BreakpointsForDimension1=V2G.WINDTURBINE.time  BeginIndexSearchUsingPreviousIndexResult=on  Table=V2G.WINDTURBINE.wind  ExtrapMethod=Clip  UseLastTableValue=on  InternalRulePriority=Speed  RndMeth=Simplest  InputSameDT=on
  Add : Sum
  Clock1 : Clock
  Constant1 : Constant
  Second-->Hour : Gain  Gain=1/3600
  " " : Outport  VectorParamsAs1DForOutWhenUnconnected=off
  wires:
  Second-->Hour/1 -> Add/1
  Add/1 -> 1-D Lookup Table/1
  Constant1/1 -> Add/2
  Clock1/1 -> Second-->Hour/1
  1-D Lookup Table/1 -> " "/1

== system simpleMicrogrid_v1/Diesel Generator/Generator Measures ==
  m : Inport
  Bus Selector : BusSelector  OutputSignals="dq0 components.Stator voltage  vq (pu),dq0 components.Stator voltage  vd (pu)"  OutputAsBus=on
  Bus Selector1 : BusSelector  OutputSignals="Mechanical.Rotor speed  wm  (pu),dq0 components.Field current  ifd (pu)"
  Fcn1 : Fcn  Expr=sqrt(u(1)^2 + u(2)^2)
  Ifd : Outport  VectorParamsAs1DForOutWhenUnconnected=off
  Vt : Outport  Port=2  VectorParamsAs1DForOutWhenUnconnected=off
  wm : Outport  Port=3  VectorParamsAs1DForOutWhenUnconnected=off
  wires:
  Bus Selector1/1 -> wm/1  "<Rotor speed  wm  (pu)>"
  m/1 -> Bus Selector1/1, Bus Selector/1
  Fcn1/1 -> Vt/1
  Bus Selector/1 -> Fcn1/1
  Bus Selector1/2 -> Ifd/1  "<Field current  ifd (pu)>"

== system simpleMicrogrid_v1/Diesel Generator/Selected Measurements ==
  m : Inport
  Bus Creator : BusCreator  Inputs=7
  Bus Selector : BusSelector  OutputSignals="Mechanical.Electrical power  Pe (pu),Mechanical.Rotor speed  wm  (pu),Output active power   Peo (pu),Output reactive power  Qeo (pu)"
  to W : Gain  Gain=Pn
  to W1 : Gain  Gain=Pn
  to W2 : Gain  Gain=Pn
  sm : Outport  VectorParamsAs1DForOutWhenUnconnected=off
  wires:
  to W2/1 -> Bus Creator/7  "Reactive Power (W)"
  to W1/1 -> Bus Creator/6  "Active Power (W)"
  Bus Selector/2 -> Bus Creator/3  "<Rotor speed  wm  (pu)>"
  Bus Creator/1 -> sm/1
  to W/1 -> Bus Creator/1  "Electrical Power (W)"
  Bus Selector/3 -> Bus Creator/4, to W1/1  "<Output active power   Peo (pu)>"
  Bus Selector/1 -> to W/1, Bus Creator/2  "<Electrical power  Pe (pu)>"
  Bus Selector/4 -> Bus Creator/5, to W2/1  "<Output reactive power  Qeo (pu)>"
  m/1 -> Bus Selector/1

== system simpleMicrogrid_v1/Energy Storage/Charge Limits ==
  SOC (%) : Inport
  Pin : Inport  Port=2
  Qin : Inport  Port=3
  Overcharge Check : Subsystem
  Undercharge Check : Subsystem
  Pbatt : Outport  VectorParamsAs1DForOutWhenUnconnected=off
  Qbatt : Outport  Port=2  VectorParamsAs1DForOutWhenUnconnected=off
  wires:
  SOC (%)/1 -> Overcharge Check/1(SOC (%)), Undercharge Check/1(SOC (%))
  Undercharge Check/2(Qout) -> Qbatt/1
  Pin/1 -> Overcharge Check/2(Pin)
  Overcharge Check/1(Pout) -> Undercharge Check/2(Pin)
  Qin/1 -> Overcharge Check/3(Qin)
  Undercharge Check/1(Pout) -> Pbatt/1  "Pbatt"
  Overcharge Check/2(Qout) -> Undercharge Check/3(Qin)

== system simpleMicrogrid_v1/Energy Storage/Reactive Power Capability ==
  Pin : Inport
  Qin : Inport  Port=2
  Constant : Constant  Value=Pnom
  Math Function : Math  Operator=square  SignedPower=on  SaturateOnIntegerOverflow=on
  Math Function1 : Math  Operator=square  SignedPower=on  SaturateOnIntegerOverflow=on
  Saturation Dynamic : simulink/Discontinuities/Saturation Dynamic  OutMin=[]  OutMax=[]  OutDataTypeStr=Inherit: Same as second input  OutDataType=fixdt(1, 16)  OutScaling=2^-10  DoSatur=off
  Sqrt : Sqrt  SaturateOnIntegerOverflow=on
  Sum : Sum  Inputs=-+|
  Unary Minus : UnaryMinus
  Qout : Outport  VectorParamsAs1DForOutWhenUnconnected=off
  wires:
  Sqrt/1 -> Saturation Dynamic/1, Unary Minus/1
  Math Function1/1 -> Sum/1
  Math Function/1 -> Sum/2
  Constant/1 -> Math Function/1
  Sum/1 -> Sqrt/1
  Unary Minus/1 -> Saturation Dynamic/3
  Saturation Dynamic/1 -> Qout/1
  Pin/1 -> Math Function1/1
  Qin/1 -> Saturation Dynamic/2

== system simpleMicrogrid_v1/Energy Storage/Stored Energy Calculation (%) ==
  Pin : Inport
  Qin : Inport  Port=2
  Charge : Gain  Gain=Efficiency/100
  Compare To Zero : simulink/Logic and Bit Operations/Compare To Zero  relop=<=  OutDataTypeStr=boolean
  Constant : Constant  Value=kWh_Rated
  Discharge : Gain  Gain=1/(Efficiency/100)
  Divide : Product  Inputs=*/
  Gain3 : Gain  Gain=1/3600/1e3
  Gain5 : Gain  Gain=-1
  Integrator : Integrator  InitialCondition=(Initial_kWh_pc/100)*kWh_Rated*3600*1e3
  Math Function1 : Math  Operator=square  SignedPower=on  SaturateOnIntegerOverflow=on
  Math Function2 : Math  Operator=square  SignedPower=on  SaturateOnIntegerOverflow=on
  Product : Product
  Sign : Signum
  Sqrt : Sqrt  SaturateOnIntegerOverflow=on
  Sum : Sum  Inputs=|++
  Switch1 : Switch  Criteria=u2 ~= 0
  Transfer Fcn : TransferFcn  Denominator=[1 1]
  to % : Gain  Gain=100
  SE% : Outport  VectorParamsAs1DForOutWhenUnconnected=off
  wires:
  Sign/1 -> Product/1
  Sqrt/1 -> Product/2
  Sum/1 -> Sqrt/1
  Math Function2/1 -> Sum/2
  Math Function1/1 -> Sum/1
  Qin/1 -> Math Function2/1
  Pin/1 -> Math Function1/1, Sign/1
  Product/1 -> Transfer Fcn/1, Discharge/1, Charge/1
  Discharge/1 -> Switch1/3
  Gain5/1 -> Integrator/1
  to %/1 -> SE%/1
  Transfer Fcn/1 -> Compare To Zero/1
  Switch1/1 -> Gain5/1
  Gain3/1 -> Divide/1
  Constant/1 -> Divide/2
  Charge/1 -> Switch1/1
  Divide/1 -> to %/1
  Compare To Zero/1 -> Switch1/2
  Integrator/1 -> Gain3/1

== system simpleMicrogrid_v1/Power Equation Wind Turbine (PQ Model)/Active Power Dynamics ==
  In : Inport
  1/Tp : Gain  Gain=1/Tp
  Integrator : Integrator
  Sum : Sum  Inputs=|+-
  Out : Outport  VectorParamsAs1DForOutWhenUnconnected=off
  wires:
  Sum/1 -> 1/Tp/1
  1/Tp/1 -> Integrator/1
  In/1 -> Sum/1
  Integrator/1 -> Sum/2, Out/1

== system simpleMicrogrid_v1/Power Equation Wind Turbine (PQ Model)/Reactive Power Dynamics ==
  In : Inport
  1/Tq : Gain  Gain=1/Tq
  Integrator : Integrator
  Sum : Sum  Inputs=|+-
  Out : Outport  VectorParamsAs1DForOutWhenUnconnected=off
  wires:
  Integrator/1 -> Out/1, Sum/2
  In/1 -> Sum/1
  1/Tq/1 -> Integrator/1
  Sum/1 -> 1/Tq/1

== system simpleMicrogrid_v1/Power Equation Wind Turbine (PQ Model)/Wind Turbine Power Equation ==
  Wind (m/s) : Inport
  Constant : Constant  Value=Pselect
  Cubic Power with Cutoff : Subsystem
  Manufacturer Fit : Lookup_n-D  NumberOfTableDimensions=1  BreakpointsForDimension1=Uvec  Table=Pvec  ExtrapMethod=Clip  InternalRulePriority=Speed  RndMeth=Simplest  InputSameDT=on
  Multiport Switch : MultiPortSwitch
  Saturation : Saturate  UpperLimit=inf  LowerLimit=0  ZeroCross=off
      settings: AttributesFormatString=|
      | %<UpperLimit>
      | %<LowerLimit>
  Wind Turbine Properties : Subsystem
  Pwind : Outport  VectorParamsAs1DForOutWhenUnconnected=off
  wires:
  Wind (m/s)/1 -> Saturation/1
  Multiport Switch/1 -> Pwind/1
  Constant/1 -> Multiport Switch/1
  Saturation/1 -> Wind Turbine Properties/1(Wind (m/s)), Manufacturer Fit/1, Cubic Power with Cutoff/1(Wind (m/s))
  Cubic Power with Cutoff/1(Pwind) -> Multiport Switch/3
  Manufacturer Fit/1 -> Multiport Switch/4
  Wind Turbine Properties/1(Pwind) -> Multiport Switch/2

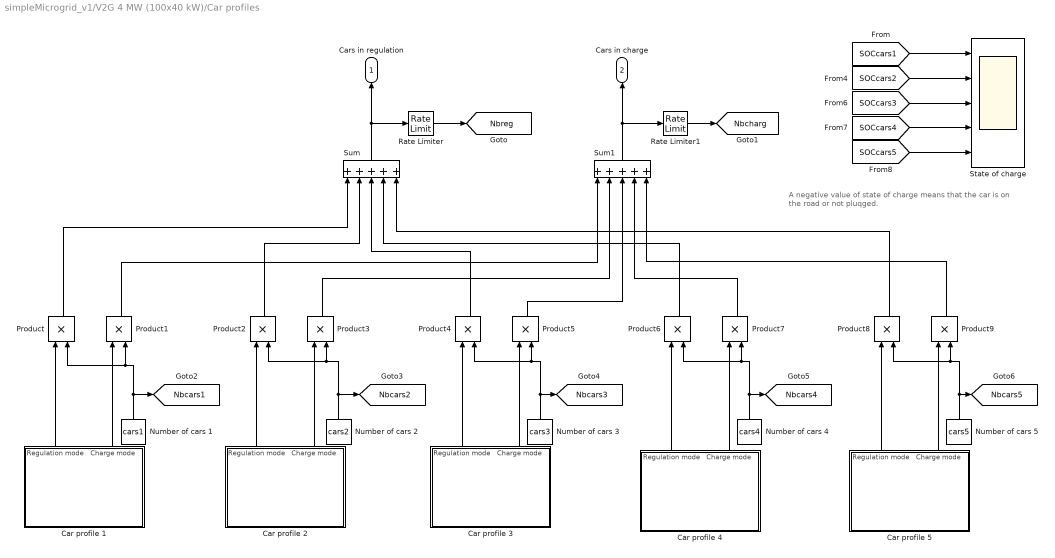
== system simpleMicrogrid_v1/V2G 4 MW (100x40 kW)/Car profiles ==
  note: A negative value of state of charge means that
      | the car is on the road or not pluqged.
  Car profile 1 : Subsystem
  Car profile 2 : Subsystem
  Car profile 3 : Subsystem
  Car profile 4 : Subsystem
  Car profile 5 : Subsystem
  Number of cars 1 : Constant  Value=cars1
  Number of cars 2 : Constant  Value=cars2
  Number of cars 3 : Constant  Value=cars3
  Number of cars 4 : Constant  Value=cars4
  Number of cars 5 : Constant  Value=cars5
  Product{,1..9} (10 alike) : Product
  Rate Limiter : RateLimiter  RisingSlewLimit=10000  FallingSlewLimit=-10000  SampleTimeMode=inherited
  Rate Limiter1 : RateLimiter  RisingSlewLimit=10000  FallingSlewLimit=-10000  SampleTimeMode=inherited
  State of charge : Scope  NumInputPorts=5
  Sum : Sum  Inputs=+++++
  Sum1 : Sum  Inputs=+++++
  Cars in regulation : Outport  VectorParamsAs1DForOutWhenUnconnected=off
  " Cars in charge" : Outport  Port=2  VectorParamsAs1DForOutWhenUnconnected=off
  tag scope: Nbcars1=global, Nbcars2=global, Nbcars3=global, Nbcars4=global, Nbcars5=global, Nbcharg=global, Nbreg=global
  wires:
  Car profile 3/2("Charge mode ") -> Product5/1
  Car profile 2/1("Regulation mode ") -> Product2/1
  Car profile 3/1("Regulation mode ") -> Product4/1
  Car profile 2/2("Charge mode ") -> Product3/1
  Car profile 4/2("Charge mode ") -> Product7/1
  Car profile 4/1("Regulation mode ") -> Product6/1
  Car profile 1/1("Regulation mode ") -> Product/1
  Car profile 1/2("Charge mode ") -> Product1/1
  Number of cars 1/1 -> [Nbcars1], Product1/2, Product/2
  Number of cars 2/1 -> [Nbcars2], Product3/2, Product2/2
  Number of cars 3/1 -> [Nbcars3], Product4/2, Product5/2
  Number of cars 4/1 -> Product6/2, Product7/2, [Nbcars4]
  Number of cars 5/1 -> Product8/2, Product9/2, [Nbcars5]
  Sum/1 -> Cars in regulation/1, Rate Limiter/1
  Sum1/1 -> Rate Limiter1/1, " Cars in charge"/1
  Product/1 -> Sum/1
  Product2/1 -> Sum/2
  Product4/1 -> Sum/3
  Product6/1 -> Sum/4
  Product8/1 -> Sum/5
  Product1/1 -> Sum1/1
  Product3/1 -> Sum1/2
  Product5/1 -> Sum1/3
  Product7/1 -> Sum1/4
  Rate Limiter/1 -> [Nbreg]
  Rate Limiter1/1 -> [Nbcharg]
  Car profile 5/1("Regulation mode ") -> Product8/1
  Car profile 5/2("Charge mode ") -> Product9/1
  Product9/1 -> Sum1/5
  [SOCcars2] -> State of charge/2
  [SOCcars3] -> State of charge/3
  [SOCcars5] -> State of charge/5
  [SOCcars4] -> State of charge/4
  [SOCcars1] -> State of charge/1

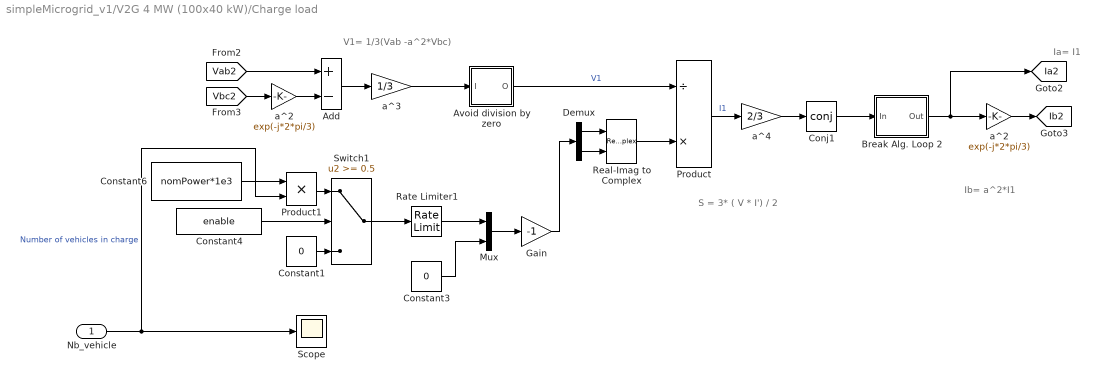
== system simpleMicrogrid_v1/V2G 4 MW (100x40 kW)/Charge load ==
  note: V1= 1/3(Vab -a^2*Vbc)
  note: S = 3* ( V * I') / 2
  note: Ia= I1
  note: Ib= a^2*I1
  Nb_vehicle : Inport
  Add : Sum  Inputs=+-
  Avoid division by zero : Subsystem
  Break Alg. Loop 2 : Subsystem
  Conj1 : Math  Operator=conj  SignedPower=on  SaturateOnIntegerOverflow=on
  Constant1 : Constant  Value=0
  Constant3 : Constant  Value=0
  Constant4 : Constant  Value=enable
  Constant6 : Constant  Value=nomPower*1e3
  Demux : Demux  Outputs=2
  Gain : Gain  Gain=-1
  Mux : Mux  Inputs=2
  Product : Product  Inputs=/*  InputSameDT=on  SaturateOnIntegerOverflow=on  OutDataTypeStr=Inherit: Same as first input
  Product1 : Product
  Rate Limiter1 : RateLimiter  RisingSlewLimit=1e4  FallingSlewLimit=-1e4  SampleTimeMode=inherited
  Real-Imag to Complex : RealImagToComplex
  Scope : Scope
  Switch1 : Switch  Threshold=0.5  ZeroCross=off
  a^2 : Gain  Gain=exp(-j*2*pi/3)  SaturateOnIntegerOverflow=on  OutDataTypeStr=Inherit: Same as input  ParamDataTypeStr=Inherit: Same as input
  "a^2 " : Gain  Gain=exp(-j*2*pi/3)  SaturateOnIntegerOverflow=on  OutDataTypeStr=Inherit: Same as input  ParamDataTypeStr=Inherit: Same as input
  a^3 : Gain  Gain=1/3  SaturateOnIntegerOverflow=on  OutDataTypeStr=Inherit: Same as input  ParamDataTypeStr=Inherit: Same as input
  a^4 : Gain  Gain=2/3  SaturateOnIntegerOverflow=on  OutDataTypeStr=Inherit: Same as input  ParamDataTypeStr=Inherit: Same as input
  tag scope: Ia2=global, Ib2=global
  wires:
  Real-Imag to Complex/1 -> Product/2
  Product/1 -> a^4/1  "I1"
  a^2/1 -> [Ib2]
  Avoid division by zero/1(O) -> Product/1  "V1"
  Conj1/1 -> Break Alg. Loop 2/1(In)
  a^3/1 -> Avoid division by zero/1(I)
  Add/1 -> a^3/1
  [Vab2] -> Add/1
  [Vbc2] -> "a^2 "/1
  "a^2 "/1 -> Add/2
  a^4/1 -> Conj1/1
  Break Alg. Loop 2/1(Out) -> [Ia2], a^2/1
  Demux/1 -> Real-Imag to Complex/1
  Demux/2 -> Real-Imag to Complex/2
  Gain/1 -> Demux/1
  Rate Limiter1/1 -> Mux/1
  Constant6/1 -> Product1/1
  Nb_vehicle/1 -> Product1/2, Scope/1  "Number of vehicles in charge"
  Constant4/1 -> Switch1/2
  Constant1/1 -> Switch1/3
  Product1/1 -> Switch1/1
  Switch1/1 -> Rate Limiter1/1
  Constant3/1 -> Mux/2
  Mux/1 -> Gain/1
